simulink library "courseFollow_cl"  (R2020a)
settings: Solver=VariableStepAuto  StartTime=0.0  StopTime=10.0  RelTol=1e-3
undefined symbols (not defined in the file or in its folder): a, pathCtrl
libraries: tanFrameProjection_ul x2, vectorNormalizer_ul x2, $bdroot x1, angleBtw2Vecs_ul x1, findClosestPointOnPath_new x1, pathGeometry_ul x1
settings Model: Creator=James Reed  LastModifiedBy=Ayaz
settings DataIOCC: ReturnWorkspaceOutputs=off
settings DebuggingCC: ArithmeticOperatorsInVariantConditions=warning
settings SFSimCC: CustomCodeUndefinedFunction=UseInterfaceOnly

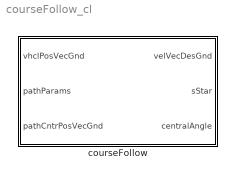
== system courseFollow_cl ==
  courseFollow : Subsystem

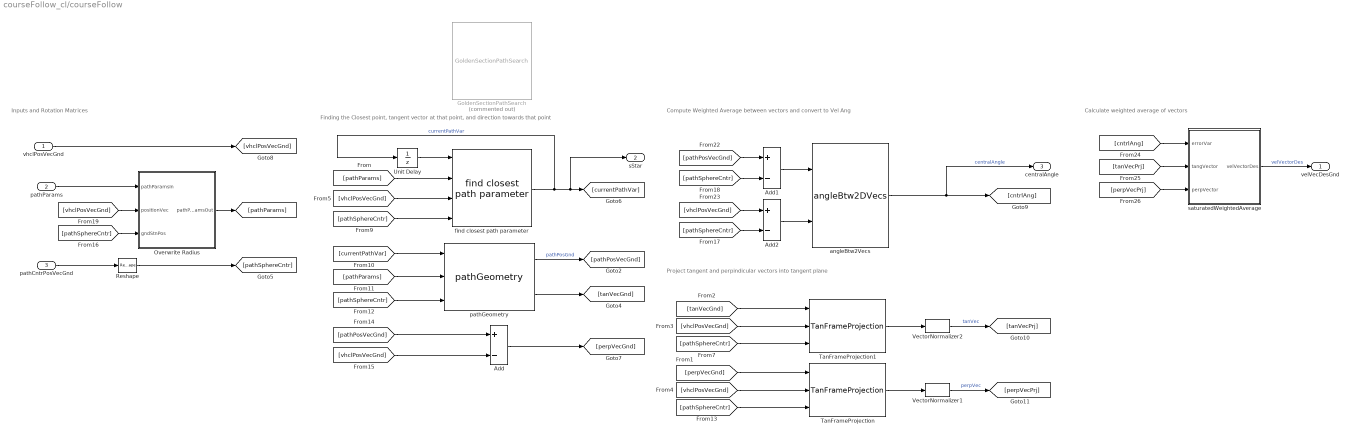
== system courseFollow_cl/courseFollow ==
  note: Calculate weighted average of vectors
  note: Project tangent and perpindicular vectors into tangent plane
  note: Compute Weighted Average between vectors and convert to Vel Ang
  note: Inputs and Rotation Matrices
  note: Finding the Closest point, tangent vector at that point, and direction towards that point
  "vhclPosVecGnd " : Inport
  pathParams : Inport  Port=2
  pathCntrPosVecGnd : Inport  Port=3
  Add : Sum  Inputs=+-
  Add1 : Sum  Inputs=+-
  Add2 : Sum  Inputs=+-
  GoldenSectionPathSearch : $bdroot/courseFollow/GoldenSectionPathSearch  Commented=on  SystemSampleTime=-1  Latency=0  AutoFrameSizeCalculation=off
  Overwrite Radius : Subsystem
  Reshape : Reshape  OutputDimensionality=Column vector (2-D)
  TanFrameProjection : tanFrameProjection_ul/TanFrameProjection  SystemSampleTime=-1  Latency=0  AutoFrameSizeCalculation=off
  TanFrameProjection1 : tanFrameProjection_ul/TanFrameProjection  SystemSampleTime=-1  Latency=0  AutoFrameSizeCalculation=off
  Unit Delay : UnitDelay  InitialCondition=pathCtrl.initPathVar.Value  SampleTime=-1  HasFrameUpgradeWarning=on
  VectorNormalizer1 : vectorNormalizer_ul/VectorNormalizer   SystemSampleTime=-1  Latency=0  AutoFrameSizeCalculation=off
  VectorNormalizer2 : vectorNormalizer_ul/VectorNormalizer   SystemSampleTime=-1  Latency=0  AutoFrameSizeCalculation=off
  angleBtw2Vecs : angleBtw2Vecs_ul/angleBtw2DVecs  SystemSampleTime=-1  Latency=0  AutoFrameSizeCalculation=off
  find closest path parameter : findClosestPointOnPath_new/find closest path parameter  maxBackward=pathCtrl.searchSize.Value/2  maxForward=pathCtrl.searchSize.Value/2  tau=0.618  convergeTol=1e-4  MaxIters=25
  pathGeometry : pathGeometry_ul/pathGeometry  SystemSampleTime=-1  Latency=0  AutoFrameSizeCalculation=off
  saturatedWeightedAverage : Subsystem  mask{error_upper_lim=pathCtrl.perpErrorVal.Value}
      mask prompts: error_upper_lim "Value of Error yielding 100% perpendicular"
  velVecDesGnd : Outport  VectorParamsAs1DForOutWhenUnconnected=off
  sStar : Outport  Port=2  VectorParamsAs1DForOutWhenUnconnected=off
  centralAngle : Outport  Port=3  VectorParamsAs1DForOutWhenUnconnected=off
  wires:
  Unit Delay/1 -> find closest path parameter/1
  [pathPosVecGnd] -> Add1/1
  VectorNormalizer2/1 -> [tanVecPrj]  "tanVec"
  [vhclPosVecGnd] -> find closest path parameter/3
  "vhclPosVecGnd "/1 -> [vhclPosVecGnd]
  pathGeometry/1 -> [pathPosVecGnd]  "pathPosGnd"
  [pathParams] -> pathGeometry/2
  VectorNormalizer1/1 -> [perpVecPrj]  "perpVec"
  angleBtw2Vecs/1 -> [cntrlAng], centralAngle/1  "centralAngle"
  [vhclPosVecGnd] -> Add2/1
  [currentPathVar] -> pathGeometry/1
  TanFrameProjection1/1 -> VectorNormalizer2/1
  [pathParams] -> find closest path parameter/2
  find closest path parameter/1 -> sStar/1, [currentPathVar], Unit Delay/1  "currentPathVar"
  Add/1 -> [perpVecGnd]
  [vhclPosVecGnd] -> Add/2
  [pathPosVecGnd] -> Add/1
  pathGeometry/2 -> [tanVecGnd]
  TanFrameProjection/1 -> VectorNormalizer1/1
  pathParams/1 -> Overwrite Radius/1(pathParamsIn)
  Overwrite Radius/1(pathParamsOut) -> [pathParams]
  pathCntrPosVecGnd/1 -> Reshape/1
  Reshape/1 -> [pathSphereCntr]
  [pathSphereCntr] -> pathGeometry/3
  [pathSphereCntr] -> find closest path parameter/4
  [pathSphereCntr] -> Add2/2
  [pathSphereCntr] -> Add1/2
  Add1/1 -> angleBtw2Vecs/1
  Add2/1 -> angleBtw2Vecs/2
  [pathSphereCntr] -> Overwrite Radius/3(gndStnPos)
  [vhclPosVecGnd] -> Overwrite Radius/2(positionVec)
  [perpVecGnd] -> TanFrameProjection/1
  [tanVecGnd] -> TanFrameProjection1/1
  [vhclPosVecGnd] -> TanFrameProjection1/2
  [vhclPosVecGnd] -> TanFrameProjection/2
  [pathSphereCntr] -> TanFrameProjection1/3
  [pathSphereCntr] -> TanFrameProjection/3
  [cntrlAng] -> saturatedWeightedAverage/1("errorVar ")
  [tanVecPrj] -> saturatedWeightedAverage/2(tangVector)
  [perpVecPrj] -> saturatedWeightedAverage/3("perpVector ")
  saturatedWeightedAverage/1("velVectorDes ") -> velVecDesGnd/1  "velVectorDes"

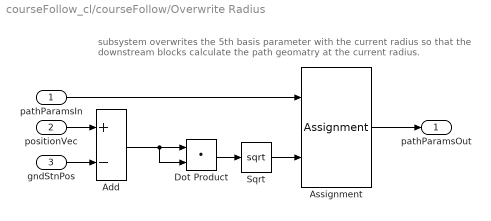
== system courseFollow_cl/courseFollow/Overwrite Radius ==
  note: subsystem overwrites the 5th basis parameter with the current radius
      | so that the downstream blocks calculate the path geomatry at the current radius.
  pathParamsIn : Inport
  positionVec : Inport  Port=2
  gndStnPos : Inport  Port=3
  Add : Sum  Inputs=+-
  Assignment : Assignment  NumberOfDimensions=2  DiagnosticForDimensions=Warning  IndexOptions=Index vector (dialog),Assign all  Indices=5,5  OutputSizes=1,1
  Dot Product : DotProduct  InputSameDT=on  OutDataTypeStr=Inherit: Inherit via internal rule
  Sqrt : Sqrt  SaturateOnIntegerOverflow=on
  pathParamsOut : Outport  VectorParamsAs1DForOutWhenUnconnected=off
  wires:
  Add/1 -> Dot Product/2, Dot Product/1
  Dot Product/1 -> Sqrt/1
  Assignment/1 -> pathParamsOut/1
  Sqrt/1 -> Assignment/2
  pathParamsIn/1 -> Assignment/1
  positionVec/1 -> Add/1
  gndStnPos/1 -> Add/2

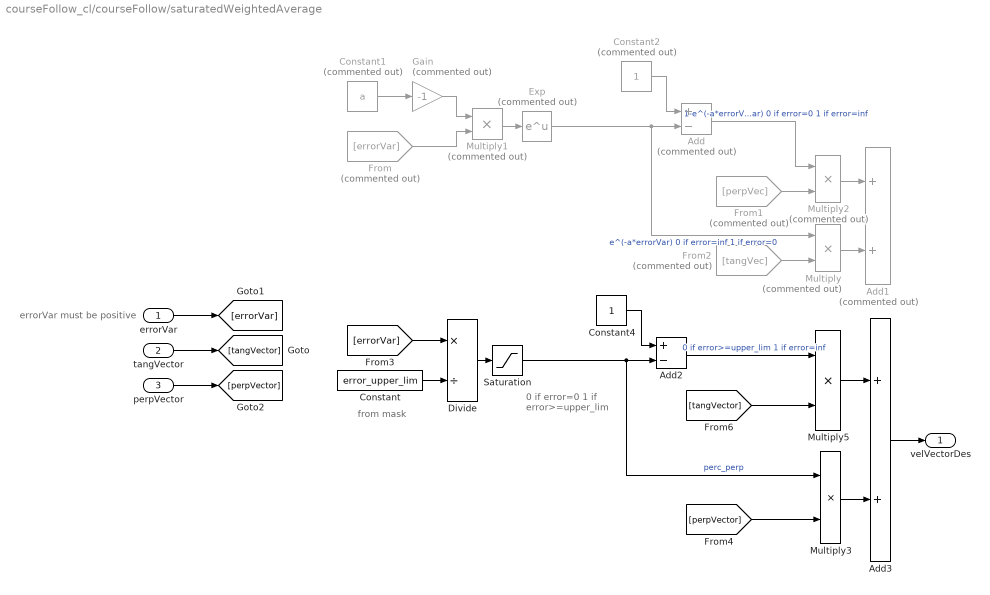
== system courseFollow_cl/courseFollow/saturatedWeightedAverage ==
  note: errorVar must be positive
  note: from mask
  note: 0 if error=0
      | 1 if error>=upper_lim
  "errorVar " : Inport
  tangVector : Inport  Port=2
  "perpVector " : Inport  Port=3
  Add : Sum  Commented=on  Inputs=+-
  Add1 : Sum  Commented=on
  Add2 : Sum  Inputs=+-
  Add3 : Sum
  Constant : Constant  Value=error_upper_lim
  Constant1 : Constant  Commented=on  Value=a
  Constant2 : Constant  Commented=on
  Constant4 : Constant
  Divide : Product  Inputs=*/
  Exp : Math  Commented=on  SignedPower=on  SaturateOnIntegerOverflow=on
  From : From  Commented=on  GotoTag=errorVar
  From1 : From  Commented=on  GotoTag=perpVec
  From2 : From  Commented=on  GotoTag=tangVec
  Gain : Gain  Commented=on  Gain=-1
  Multiply : Product  Commented=on
  Multiply1 : Product  Commented=on
  Multiply2 : Product  Commented=on
  Multiply3 : Product
  Multiply5 : Product
  Saturation : Saturate  UpperLimit=1  LowerLimit=0
  "velVectorDes " : Outport  VectorParamsAs1DForOutWhenUnconnected=off
  wires:
  [perpVector] -> Multiply3/2
  [tangVector] -> Multiply5/2
  Divide/1 -> Saturation/1
  Constant/1 -> Divide/2
  [errorVar] -> Divide/1
  Add2/1 -> Multiply5/1  "0 if error>=upper_lim 1 if error=inf"
  Multiply5/1 -> Add3/1
  Multiply3/1 -> Add3/2
  Add3/1 -> "velVectorDes "/1
  Saturation/1 -> Add2/2, Multiply3/1  "perc_perp"
  Constant4/1 -> Add2/1
  From2/1 -> Multiply/2
  From1/1 -> Multiply2/2
  Multiply/1 -> Add1/2
  Multiply2/1 -> Add1/1
  From/1 -> Multiply1/2
  "perpVector "/1 -> [perpVector]
  "errorVar "/1 -> [errorVar]
  Add/1 -> Multiply2/1  "1-e^(-a*errorVar) 0 if error=0 1 if error=inf"
  Constant2/1 -> Add/1
  Exp/1 -> Add/2, Multiply/1  "e^(-a*errorVar) 0 if error=inf 1 if error=0"
  Multiply1/1 -> Exp/1
  Gain/1 -> Multiply1/1
  Constant1/1 -> Gain/1
  tangVector/1 -> [tangVector]
